simulink model "done_with_heading_and_directional_autopilot"  (R2019a)
settings: Solver=VariableStepAuto  StartTime=0.0  StopTime=2000  RelTol=1e-3
values from neighbouring files (symbols this model uses):
  A = [-0.0804 0.1665 0 -9.8100 0 ... (first row only)    [longitudinaloia.m]    (also in oia.m = [-0.1245 0.0350 0.0414 -0.9962 0; -15.2138 -2.0587 0.0032 0.; state_space2tf.m = [-0.0558 -0.9968 0.0802 0.0415;0.5980 -0.1150 -0.0318 0;-3.0)
  B = [0 32.1224 ... (first row only)    [longitudinaloia.m]    (also in oia.m = [-0.0049 0.0237 ;-4.0379 0.9613; 0   0  ; -0.0568 -1.2168; 0; state_space2tf.m = [0.0073 0; -0.4750    0.0077;  0.1530    0.1430;0         0])
  C = [1          0          0          0 0;  0          1       0          0 0 ; 0       0          1          0 0; 0  0    0        1 0; 0 0 0 0 1]    [longitudinaloia.m]    (also in oia.m; state_space2tf.m = [0     1     0     0;  0     0     0     1])
  D = [0 0 ;0 0 ; 0 0 ;0   0;0 0]    [longitudinaloia.m]    (also in oia.m; state_space2tf.m = [0 0; 0 0])
settings Model: Creator=admin  LastModifiedBy=admin

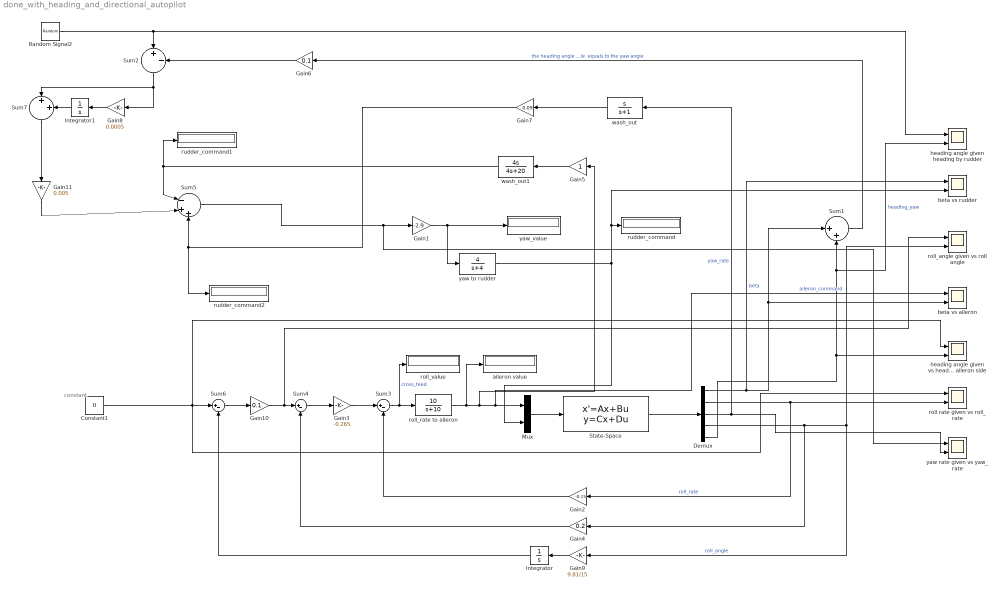
== system done_with_heading_and_directional_autopilot ==
  note: constant
  Constant1 : Constant  Value=0
  Demux : Demux  Outputs=5
  Gain1 : Gain  Gain=-2.9
  Gain10 : Gain  Gain=0.1
  Gain11 : Gain  Gain=0.005
  Gain2 : Gain  Gain=-0.15
  Gain3 : Gain  Gain=-0.265
  Gain4 : Gain  Gain=0.2
  Gain5 : Gain
  Gain6 : Gain  Gain=0.1
  Gain7 : Gain  Gain=0.09
  Gain8 : Gain  Gain=0.0005
  Gain9 : Gain  Gain=9.81/15
  Integrator : Integrator
  Integrator1 : Integrator
  Mux : Mux  Inputs=2
  Random Signal2 : RandomNumber  SampleTime=50
  State-Space : StateSpace  A=A  B=B  C=C  D=D  InitialCondition=[0.5,0.75,0.4,0.2,0.1]
  Sum1 : Sum  Inputs=|++
  Sum{2..4,6} (4 alike) : Sum  Inputs=|+-
  Sum5 : Sum  Inputs=|-++
  Sum7 : Sum  Inputs=|++
  aileron value : Display
  beta vs aileron : Scope  NumInputPorts=2
  beta vs rudder : Scope  NumInputPorts=2
  heading angle given heading by rudder : Scope  NumInputPorts=2
  heading angle given vs heading_angle/yaw by aileron side : Scope  NumInputPorts=2
  "roll rate given vs roll_rate " : Scope  NumInputPorts=2
  roll_angle given vs roll angle : Scope  NumInputPorts=2
  roll_rate to aileron : TransferFcn  Numerator=[10]  Denominator=[1 10]
  roll_value : Display
  rudder_command : Display
  rudder_command1 : Display
  rudder_command2 : Display
  wash_out : TransferFcn  Numerator=[1 0]  Denominator=[1 1]
  wash_out1 : TransferFcn  Numerator=[4 0]  Denominator=[4 20]
  "yaw rate given vs yaw_rate " : Scope  NumInputPorts=2
  yaw to rudder : TransferFcn  Numerator=[4]  Denominator=[1 4]
  yaw_value : Display
  wires:
  Mux/1 -> State-Space/1
  State-Space/1 -> Demux/1
  Demux/1 -> beta vs rudder/1, Sum1/1, beta vs aileron/2  "beta"
  Demux/2 -> Gain2/1, "roll rate given vs roll_rate "/2  "roll_rate"
  Demux/3 -> "yaw rate given vs yaw_rate "/2, wash_out/1  "yaw_rate"
  Demux/4 -> Gain9/1, roll_angle given vs roll angle/2, Gain4/1  "roll_angle"
  Demux/5 -> heading angle given heading by rudder/2, Sum1/2, heading angle given vs heading_angle/yaw by aileron side/2  "heading_yaw"
  roll_rate to aileron/1 -> aileron value/1, beta vs aileron/1, Mux/1, Gain5/1  "aileron_command"
  Sum3/1 -> roll_value/1, roll_rate to aileron/1  "cross_feed"
  Gain2/1 -> Sum3/2
  Sum4/1 -> Gain3/1
  Gain3/1 -> Sum3/1
  Gain4/1 -> Sum4/2
  wash_out/1 -> Gain7/1
  Sum5/1 -> "yaw rate given vs yaw_rate "/1, Gain1/1
  yaw to rudder/1 -> beta vs rudder/2, rudder_command/1, Mux/2
  Gain5/1 -> wash_out1/1
  Gain1/1 -> yaw to rudder/1, yaw_value/1
  Gain7/1 -> rudder_command2/1, Sum5/3
  wash_out1/1 -> Sum5/1, rudder_command1/1
  Constant1/1 -> Sum6/1, "roll rate given vs roll_rate "/1, heading angle given vs heading_angle/yaw by aileron side/1
  Integrator/1 -> Sum6/2
  Gain9/1 -> Integrator/1
  Gain10/1 -> roll_angle given vs roll angle/1, Sum4/1
  Sum6/1 -> Gain10/1
  Sum1/1 -> Gain6/1  "the heading angle lamda is given by (beta + yaw angle) essentially when beta is zero heading angle  equals to the yaw angle"
  Random Signal2/1 -> heading angle given heading by rudder/1, Sum2/1
  Gain6/1 -> Sum2/2
  Sum2/1 -> Gain8/1, Sum7/1
  Integrator1/1 -> Sum7/2
  Gain8/1 -> Integrator1/1
  Sum7/1 -> Gain11/1
  Gain11/1 -> Sum5/2
